simulink model "CruiseControl_SwArch"  (R2021b)
settings: Solver=FixedStepDiscrete  StartTime=0.0  StopTime=10.0  RelTol=1e-3
model workspace (MAT data in the model file):
  BrakePosition = Simulink.ValueType
  CruiseCtrlCmds = Simulink.Bus
  CruiseCtrlCmds.Alignment = -1
  CruiseCtrlCmds.PreserveElementDimensions = 0
  CruiseCtrlCmds.Elements_internal(1) = Simulink.BusElement
  CruiseCtrlCmds.Elements_internal(1).DimensionsMode = 'Fixed'
  CruiseCtrlCmds.Elements_internal(1).SamplingMode = 'Sample based'
  CruiseCtrlCmds.Elements_internal(1).SampleTime = -1
  CruiseCtrlCmds.Elements_internal(1).Name = 'CruiseButton'
  CruiseCtrlCmds.Elements_internal(1).DataType_internal = 'boolean'
  CruiseCtrlCmds.Elements_internal(1).Complexity = 'real'
  CruiseCtrlCmds.Elements_internal(1).Dimensions = 1
  CruiseCtrlCmds.Elements_internal(2) = Simulink.BusElement
  CruiseCtrlCmds.Elements_internal(2).DimensionsMode = 'Fixed'
  CruiseCtrlCmds.Elements_internal(2).SamplingMode = 'Sample based'
  CruiseCtrlCmds.Elements_internal(2).SampleTime = -1
  CruiseCtrlCmds.Elements_internal(2).Name = 'CancelButton'
  CruiseCtrlCmds.Elements_internal(2).DataType_internal = 'boolean'
  CruiseCtrlCmds.Elements_internal(2).Complexity = 'real'
  CruiseCtrlCmds.Elements_internal(2).Dimensions = 1
  CruiseCtrlCmds.Elements_internal(3) = Simulink.BusElement
  CruiseCtrlCmds.Elements_internal(3).DimensionsMode = 'Fixed'
  CruiseCtrlCmds.Elements_internal(3).SamplingMode = 'Sample based'
  CruiseCtrlCmds.Elements_internal(3).SampleTime = -1
  CruiseCtrlCmds.Elements_internal(3).Name = 'SetButton'
  CruiseCtrlCmds.Elements_internal(3).DataType_internal = 'boolean'
  CruiseCtrlCmds.Elements_internal(3).Complexity = 'real'
  CruiseCtrlCmds.Elements_internal(3).Dimensions = 1
  CruiseCtrlCmds.Elements_internal(4) = Simulink.BusElement
  CruiseCtrlCmds.Elements_internal(4).DimensionsMode = 'Fixed'
  CruiseCtrlCmds.Elements_internal(4).SamplingMode = 'Sample based'
  CruiseCtrlCmds.Elements_internal(4).SampleTime = -1
  CruiseCtrlCmds.Elements_internal(4).Name = 'ResumeButton'
  CruiseCtrlCmds.Elements_internal(4).DataType_internal = 'boolean'
  CruiseCtrlCmds.Elements_internal(4).Complexity = 'real'
  CruiseCtrlCmds.Elements_internal(4).Dimensions = 1
  CruiseCtrlCmds.Elements_internal(5) = Simulink.BusElement
  CruiseCtrlCmds.Elements_internal(5).DimensionsMode = 'Fixed'
  CruiseCtrlCmds.Elements_internal(5).SamplingMode = 'Sample based'
  CruiseCtrlCmds.Elements_internal(5).SampleTime = -1
  CruiseCtrlCmds.Elements_internal(5).Name = 'IncrementButton'
  CruiseCtrlCmds.Elements_internal(5).DataType_internal = 'boolean'
  CruiseCtrlCmds.Elements_internal(5).Complexity = 'real'
  CruiseCtrlCmds.Elements_internal(5).Dimensions = 1
  CruiseCtrlCmds.Elements_internal(6) = Simulink.BusElement
  CruiseCtrlCmds.Elements_internal(6).DimensionsMode = 'Fixed'
  CruiseCtrlCmds.Elements_internal(6).SamplingMode = 'Sample based'
  CruiseCtrlCmds.Elements_internal(6).SampleTime = -1
  CruiseCtrlCmds.Elements_internal(6).Name = 'DecrementButton'
  CruiseCtrlCmds.Elements_internal(6).DataType_internal = 'boolean'
  CruiseCtrlCmds.Elements_internal(6).Complexity = 'real'
  CruiseCtrlCmds.Elements_internal(6).Dimensions = 1
  CruiseCtrlCmds.DataScope = 'Auto'
  CruiseCtrlMode = Simulink.ValueType
  CruiseCtrlMode.DataType = 'int32'
  DriverRequest = Simulink.ValueType
  DriverRequest.DataType = 'int32'
  GearPosition = Simulink.ValueType
  GearPosition.DataType = 'int32'
  Indicators = Simulink.Bus
  Indicators.Alignment = -1
  Indicators.PreserveElementDimensions = 0
  Indicators.Elements_internal(1) = Simulink.BusElement
  Indicators.Elements_internal(1).DimensionsMode = 'Fixed'
  Indicators.Elements_internal(1).SamplingMode = 'Sample based'
  Indicators.Elements_internal(1).SampleTime = -1
  Indicators.Elements_internal(1).Name = 'CruiseIndicator'
  Indicators.Elements_internal(1).DataType_internal = 'boolean'
  Indicators.Elements_internal(1).Complexity = 'real'
  Indicators.Elements_internal(1).Dimensions = 1
  Indicators.Elements_internal(2) = Simulink.BusElement
  Indicators.Elements_internal(2).DimensionsMode = 'Fixed'
  Indicators.Elements_internal(2).SamplingMode = 'Sample based'
  Indicators.Elements_internal(2).SampleTime = -1
  Indicators.Elements_internal(2).Name = 'SetIndicator'
  Indicators.Elements_internal(2).DataType_internal = 'boolean'
  Indicators.Elements_internal(2).Complexity = 'real'
  Indicators.Elements_internal(2).Dimensions = 1
  Indicators.DataScope = 'Auto'
  KeyPosition = Simulink.ValueType
  KeyPosition.DataType = 'int32'
  TargetSpeed = Simulink.ValueType
  ThrottleCmd = Simulink.ValueType
  ThrottleValue = Simulink.ValueType
  VehicleSpeed = Simulink.ValueType
settings Model: Creator=rsnah  LastModifiedBy=rsnah

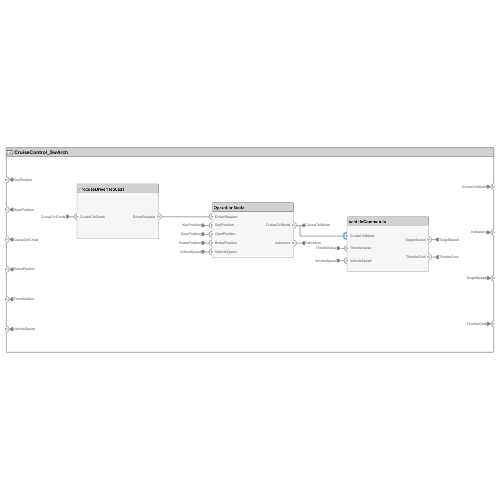
[thumbnail: Simulink's stored preview of the top-level diagram]
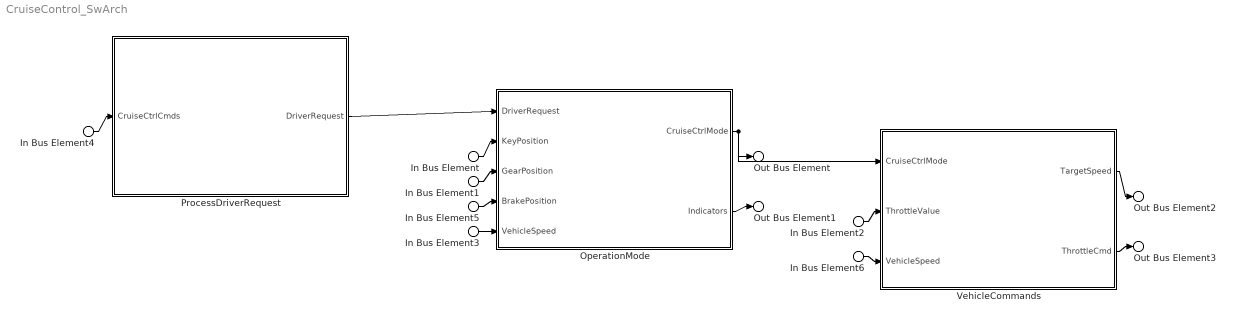
== system CruiseControl_SwArch ==
  In Bus Element : Inport  PortName=KeyPosition
  In Bus Element1 : Inport  Port=2  PortName=GearPosition
  In Bus Element4 : Inport  Port=3  PortName=CruiseCtrlCmds
  In Bus Element5 : Inport  Port=4  PortName=BrakePosition
  In Bus Element2 : Inport  Port=5  PortName=ThrottleValue
  In Bus Element3 : Inport  Port=6  PortName=VehicleSpeed
  In Bus Element6 : Inport  Port=6  PortName=VehicleSpeed
  OperationMode : Subsystem
      settings: PortSchema="{\"entries\":[{\"content\":{\"headerSize\":26,\"margin\":15,\"minimumSpacing\":25,\"sides\":[{\"content\":{\"connectorIds\":[\"In2\",\"In3\",\"In4\",\"In5\",\"In1\"]},\"type\":\"ConnectorPlacement.EquallySpacedRectSide\",\"uuid\":\"9f07c548-25e4-482a-abb8-5e8bc29b591a\"},{\"content\":{\"connectorIds\":[\"Out1\",\"Out2\"],\"side\":\"RIGHT\"},\"type\":\"ConnectorPlacement.EquallySpacedRectSide\",\"uuid\":\"1e04a542-a681-42e8-a716-8d6bb79a3186\"},{\"content\":{\"connectorIds\":[],\"side\":\"TOP\"},\"type\":\"ConnectorPlacement.EquallySpacedRectSide\",\"uuid\":\"95d5d46a-b390-4de2-bab2-f1971cad08b9\"},{\"content\":{\"connectorIds\":[],\"side\":\"BOTTOM\"},\"type\":\"ConnectorPlacement.EquallySpacedRectSide\",\"uuid\":\"c03020ac-14fd-4a69-b274-38089dd50528\"}]},\"type\":\"ConnectorPlacement.EquallySpacedConnector\",\"uuid\":\"6cc3ec22-7ae2-45b3-bcd1-e43dff26b2ac\"}],\"packageUris\":[\"http://schema.mathworks.com/mf0/Connector/R2020b\"],\"version\":\"1.0\"}"
  ProcessDriverRequest : Subsystem
      settings: PortSchema="{\"entries\":[{\"content\":{\"headerSize\":26,\"margin\":15,\"minimumSpacing\":25,\"sides\":[{\"content\":{\"connectorIds\":[\"In1\"]},\"type\":\"ConnectorPlacement.EquallySpacedRectSide\",\"uuid\":\"9f07c548-25e4-482a-abb8-5e8bc29b591a\"},{\"content\":{\"connectorIds\":[\"Out1\"],\"side\":\"RIGHT\"},\"type\":\"ConnectorPlacement.EquallySpacedRectSide\",\"uuid\":\"1e04a542-a681-42e8-a716-8d6bb79a3186\"},{\"content\":{\"connectorIds\":[],\"side\":\"TOP\"},\"type\":\"ConnectorPlacement.EquallySpacedRectSide\",\"uuid\":\"95d5d46a-b390-4de2-bab2-f1971cad08b9\"}]},\"type\":\"ConnectorPlacement.EquallySpacedConnector\",\"uuid\":\"6cc3ec22-7ae2-45b3-bcd1-e43dff26b2ac\"}],\"packageUris\":[\"http://schema.mathworks.com/mf0/Connector/R2020b\"],\"version\":\"1.0\"}"
  VehicleCommands : Subsystem
      settings: PortSchema="{\"entries\":[{\"content\":{\"headerSize\":26,\"margin\":15,\"minimumSpacing\":25,\"sides\":[{\"content\":{\"connectorIds\":[\"In1\",\"In2\",\"In3\"]},\"type\":\"ConnectorPlacement.EquallySpacedRectSide\",\"uuid\":\"9f07c548-25e4-482a-abb8-5e8bc29b591a\"},{\"content\":{\"connectorIds\":[\"Out1\",\"Out2\"],\"side\":\"RIGHT\"},\"type\":\"ConnectorPlacement.EquallySpacedRectSide\",\"uuid\":\"1e04a542-a681-42e8-a716-8d6bb79a3186\"},{\"content\":{\"connectorIds\":[],\"side\":\"TOP\"},\"type\":\"ConnectorPlacement.EquallySpacedRectSide\",\"uuid\":\"95d5d46a-b390-4de2-bab2-f1971cad08b9\"}]},\"type\":\"ConnectorPlacement.EquallySpacedConnector\",\"uuid\":\"6cc3ec22-7ae2-45b3-bcd1-e43dff26b2ac\"}],\"packageUris\":[\"http://schema.mathworks.com/mf0/Connector/R2020b\"],\"version\":\"1.0\"}"
  Out Bus Element : Outport  PortName=CruiseCtrlMode
  Out Bus Element1 : Outport  Port=2  PortName=Indicators
  Out Bus Element2 : Outport  Port=3  PortName=TargetSpeed
  Out Bus Element3 : Outport  Port=4  PortName=ThrottleCmd
  wires:
  In Bus Element/1 -> OperationMode/3(KeyPosition)
  In Bus Element1/1 -> OperationMode/4(GearPosition)
  In Bus Element5/1 -> OperationMode/5(BrakePosition)
  In Bus Element3/1 -> OperationMode/1(VehicleSpeed)
  OperationMode/2(Indicators) -> Out Bus Element1/1
  In Bus Element2/1 -> VehicleCommands/2(ThrottleValue)
  In Bus Element6/1 -> VehicleCommands/3(VehicleSpeed)
  OperationMode/1(CruiseCtrlMode) -> Out Bus Element/1, VehicleCommands/1(CruiseCtrlMode)
  In Bus Element4/1 -> ProcessDriverRequest/1(CruiseCtrlCmds)
  ProcessDriverRequest/1(DriverRequest) -> OperationMode/2(DriverRequest)
  VehicleCommands/1(TargetSpeed) -> Out Bus Element2/1
  VehicleCommands/2(ThrottleCmd) -> Out Bus Element3/1

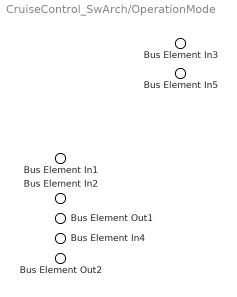
== system CruiseControl_SwArch/OperationMode ==
  Bus Element In5 : Inport  PortName=VehicleSpeed
  Bus Element In3 : Inport  Port=2  PortName=DriverRequest
  Bus Element In1 : Inport  Port=3  PortName=KeyPosition
  Bus Element In2 : Inport  Port=4  PortName=GearPosition
  Bus Element In4 : Inport  Port=5  PortName=BrakePosition
  Bus Element Out1 : Outport  PortName=CruiseCtrlMode
  Bus Element Out2 : Outport  Port=2  PortName=Indicators

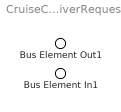
== system CruiseControl_SwArch/ProcessDriverRequest ==
  Bus Element In1 : Inport  PortName=CruiseCtrlCmds
  Bus Element Out1 : Outport  PortName=DriverRequest

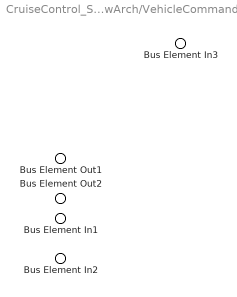
== system CruiseControl_SwArch/VehicleCommands ==
  Bus Element In3 : Inport  PortName=CruiseCtrlMode
  Bus Element In1 : Inport  Port=2  PortName=ThrottleValue
  Bus Element In2 : Inport  Port=3  PortName=VehicleSpeed
  Bus Element Out1 : Outport  PortName=TargetSpeed
  Bus Element Out2 : Outport  Port=2  PortName=ThrottleCmd
